simulink model "final_com_observer"  (R2017a)
settings: Solver=VariableStepAuto  StartTime=0.0  StopTime=15  RelTol=1e-3
values from neighbouring files (symbols this model uses):
  L = place (A',C',J_obs)    [principal.m]
undefined symbols (not defined in the file or in its folder): K_lqr
libraries: simulink x6
settings Model: Creator=dscat  LastModifiedBy=dscat

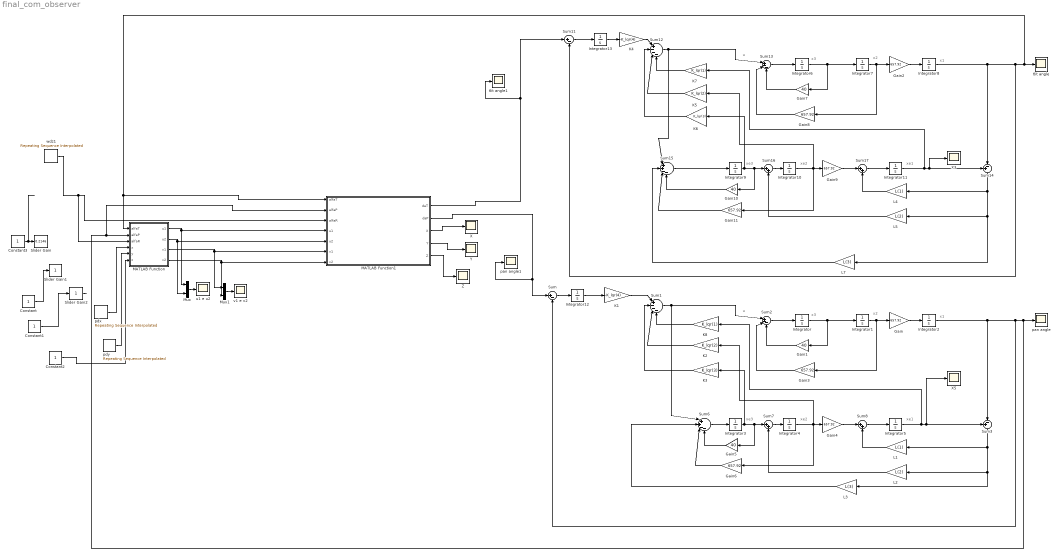
== system final_com_observer ==
  note: x2
  note: u
  note: xe1
  note: x1
  note: x3
  note: xe3
  note: xe2
  note: x2
  note: u
  note: xe1
  note: x1
  note: x3
  note: xe3
  note: xe2
  Constant{,1..3} (4 alike) : Constant
  Gain{,2..4,6,8..9,11} (8 alike) : Gain  Gain=657.92
  Gain{1,5,7,10} (4 alike) : Gain  Gain=40
  Integrator{,1..13} (14 alike) : Integrator
  K1 : Gain  Gain=-K_lqr(4)
  K2 : Gain  Gain=K_lqr(2)
  K3 : Gain  Gain=K_lqr(3)
  K4 : Gain  Gain=-K_lqr(4)
  K5 : Gain  Gain=K_lqr(2)
  K6 : Gain  Gain=K_lqr(3)
  K7 : Gain  Gain=K_lqr(1)
  K8 : Gain  Gain=K_lqr(1)
  L1 : Gain  Gain=L(1)
  L2 : Gain  Gain=L(2)
  L3 : Gain  Gain=L(3)
  L4 : Gain  Gain=L(1)
  L5 : Gain  Gain=L(2)
  L7 : Gain  Gain=L(3)
  MATLAB Function : MATLAB Function  TreatAsAtomicUnit=on
  MATLAB Function1 : MATLAB Function  TreatAsAtomicUnit=on
  Mux : Mux  Inputs=2
  Mux1 : Mux  Inputs=2
  Slider Gain : simulink/Math Operations/Slider Gain  gain=0.2146  low=-3.14  high=3.14
  Slider Gain1 : simulink/Math Operations/Slider Gain  gain=1  low=-5  high=5
  Slider Gain2 : simulink/Math Operations/Slider Gain  gain=1  low=-5  high=5
  Sum : Sum  Inputs=|+-
  Sum1 : Sum  Inputs=|+---
  Sum11 : Sum  Inputs=|+-
  Sum12 : Sum  Inputs=|+---
  Sum13 : Sum  Inputs=|+--
  Sum14 : Sum  Inputs=+-|
  Sum15 : Sum  Inputs=|++--
  Sum{7..8,16..17} (4 alike) : Sum  Inputs=|++
  Sum2 : Sum  Inputs=|+--
  Sum3 : Sum  Inputs=+-|
  Sum6 : Sum  Inputs=|++--
  X : Scope
  X3 : Scope
  X5 : Scope
  Y : Scope
  Z : Scope
  pan angle : Scope
  pan angle1 : Scope
  pdx : simulink/Sources/Repeating Sequence Interpolated  OutValues=pdx  TimeValues=t  LookUpMeth=Interpolation-Use End Values  tsamp=0.01  OutMin=[]  OutMax=[]  OutDataTypeStr=double  OutputDataTypeScalingMode=double  OutDataType=fixdt(0,8)  OutScaling=2^-10
  pdy : simulink/Sources/Repeating Sequence Interpolated  OutValues=pdy  TimeValues=t  LookUpMeth=Interpolation-Use End Values  tsamp=0.01  OutMin=[]  OutMax=[]  OutDataTypeStr=double  OutputDataTypeScalingMode=double  OutDataType=fixdt(0,8)  OutScaling=2^-10
  tlit angle : Scope
  tlit angle1 : Scope
  u1 e u2 : Scope
  v1 e v2 : Scope
  wdz1 : simulink/Sources/Repeating Sequence Interpolated  OutValues=wdz  TimeValues=t  LookUpMeth=Interpolation-Use End Values  tsamp=0.01  OutMin=[]  OutMax=[]  OutDataTypeStr=double  OutputDataTypeScalingMode=double  OutDataType=fixdt(0,8)  OutScaling=2^-10
  wires:
  MATLAB Function1/3(X) -> X/1
  MATLAB Function1/4(Y) -> Y/1
  MATLAB Function1/5(Z) -> Z/1
  Integrator8/1 -> Sum14/2, Sum11/2, tlit angle/1, MATLAB Function1/1(alfaT), MATLAB Function/1(alfaT)
  Integrator2/1 -> Sum3/2, Sum/2, pan angle/1, MATLAB Function1/2(alfaP), MATLAB Function/2(alfaP)
  Constant3/1 -> Slider Gain/1
  Constant1/1 -> Slider Gain2/1
  Mux1/1 -> v1 e v2/1
  Mux/1 -> u1 e u2/1
  Constant/1 -> Slider Gain1/1
  MATLAB Function/4(v2) -> MATLAB Function1/7(v2), Mux1/2
  MATLAB Function/1(u1) -> MATLAB Function1/4(u1), Mux/1
  MATLAB Function/3(v1) -> MATLAB Function1/6(v1), Mux1/1
  MATLAB Function/2(u2) -> MATLAB Function1/5(u2), Mux/2
  Gain5/1 -> Sum6/4
  Sum8/1 -> Integrator5/1
  Integrator4/1 -> K2/1, Gain6/1, Gain4/1
  L2/1 -> Sum7/2
  Sum7/1 -> Integrator4/1
  Gain4/1 -> Sum8/1
  Integrator3/1 -> Sum7/1, Gain5/1, K3/1
  K3/1 -> Sum1/2
  Sum/1 -> Integrator12/1
  L1/1 -> Sum8/2
  Gain6/1 -> Sum6/3
  Gain1/1 -> Sum2/3
  Integrator5/1 -> K8/1, X5/1, Sum3/1
  Gain3/1 -> Sum2/2
  L3/1 -> Sum6/2
  Sum3/1 -> L1/1, L2/1, L3/1
  MATLAB Function1/2(daP) -> pan angle1/1, Sum/1
  Integrator/1 -> Gain1/1, Integrator1/1
  Sum6/1 -> Integrator3/1
  Gain/1 -> Integrator2/1
  Integrator1/1 -> Gain3/1, Gain/1
  K2/1 -> Sum1/3
  Sum1/1 -> Sum2/1, Sum6/1
  Sum2/1 -> Integrator/1
  K1/1 -> Sum1/1
  Gain10/1 -> Sum15/4
  Sum17/1 -> Integrator11/1
  Integrator10/1 -> K5/1, Gain11/1, Gain9/1
  L5/1 -> Sum16/2
  Sum16/1 -> Integrator10/1
  Gain9/1 -> Sum17/1
  Integrator9/1 -> Sum16/1, Gain10/1, K6/1
  K6/1 -> Sum12/2
  Sum11/1 -> Integrator13/1
  L4/1 -> Sum17/2
  Gain11/1 -> Sum15/3
  Gain7/1 -> Sum13/3
  Integrator11/1 -> K7/1, X3/1, Sum14/1
  Gain8/1 -> Sum13/2
  Sum14/1 -> L4/1, L5/1, L7/1
  Integrator6/1 -> Gain7/1, Integrator7/1
  Gain2/1 -> Integrator8/1
  Integrator7/1 -> Gain8/1, Gain2/1
  K5/1 -> Sum12/3
  Sum12/1 -> Sum13/1, Sum15/1
  Sum13/1 -> Integrator6/1
  K4/1 -> Sum12/1
  Integrator13/1 -> K4/1
  K7/1 -> Sum12/4
  Sum15/1 -> Integrator9/1
  L7/1 -> Sum15/2
  K8/1 -> Sum1/4
  MATLAB Function1/1(daT) -> Sum11/1, tlit angle1/1
  Constant2/1 -> MATLAB Function/6(z)
  Integrator12/1 -> K1/1
  wdz1/1 -> MATLAB Function1/3(alfaR), MATLAB Function/3(alfaR)
  Slider Gain2/1 -> ?
  pdx/1 -> MATLAB Function/4(x)
  pdy/1 -> MATLAB Function/5(y)

== matlab function final_com_observer/MATLAB Function1 ==
  data: alfaT input; daT output; alfaP input; alfaR input; u1 input; u2 input; v1 input; v2 input; daP output; X output; Y output; Z output
function [daT, daP, X,Y,Z  ] = image2real( alfaT,alfaP,alfaR, u1,u2,v1,v2)
% daT -> Delta Alfa Tilt
% daP -> Delta Alfa Pan
% AlfaR -> Lido dos encoders


l = 0.15; %Tamanho do alvo (m) 
f = 664;

X = (l*(f*cos(alfaP-alfaR) - u2*sin(alfaP-alfaR))*(- cos(alfaP-alfaR)*sin(alfaP-alfaR)*f^2 + (u1 - cos(alfaP-alfaR)^2*(u1 + u2))*f + u1*u2*cos(alfaP-alfaR)*sin(alfaP-alfaR)))/(f*(u2*cos(alfaP-alfaR) + f*sin(alfaP-alfaR))*(u1 - u2));

%X = (l*(f*cos(alfaT) - v2*sin(alfaT))*(- cos(alfaT)*sin(alfaT)*f^2 + (v1 - cos(alfaT)^2*(v1 + v2))*f + v1*v2*cos(alfaT)*sin(alfaT)))/(f*(f*sin(alfaT) + v2*cos(alfaT))*(v1 - v2));

Y = -(l*(2*cos(alfaP-alfaR)*sin(alfaP-alfaR)*f^2 + (u1 + u2)*(2*cos(alfaP-alfaR)^2 - 1)*f - 2*u1*u2*cos(alfaP-alfaR)*sin(alfaP-alfaR)))/(2*f*(u1 - u2));

Z  = -(l*(2*cos(alfaT)*sin(alfaT)*f^2 + (v1 + v2)*(2*cos(alfaT)^2 - 1)*f - 2*v1*v2*cos(alfaT)*sin(alfaT)))/(2*f*(v1 - v2));
 
daP = double(atan(Y/X)+alfaR);
%daT = double(atan(Z/(sqrt((X)^2+(Y)^2))));
daT = double(atan(Z/X));

end

== matlab function final_com_observer/MATLAB Function ==
  data: alfaT input; u1 output; alfaP input; alfaR input; x input; y input; z input; u2 output; v1 output; v2 output
function [u1, u2, v1, v2] = real2image(alfaT,alfaP,alfaR,x,y,z)
L = 0.15;
f = 664;
u1 = f*(-sin(alfaP-alfaR)*(-x)+cos(alfaP-alfaR)*((L/2)-y))/((cos(alfaP-alfaR)*(-x)+sin(alfaP-alfaR)*((L/2)-y)));
u2 = f*(-sin(alfaP-alfaR)*(-x)+cos(alfaP-alfaR)*((-L/2)-y))/((cos(alfaP-alfaR)*(-x)+sin(alfaP-alfaR)*((-L/2)-y)));
v1 = f*(-sin(alfaT)*(-x)+cos(alfaT)*((L/2)-z))/((cos(alfaT)*(-x)+sin(alfaT)*((L/2)-z)));
v2 = f*(-sin(alfaT)*(-x)+cos(alfaT)*((-L/2)-z))/((cos(alfaT)*(-x)+sin(alfaT)*((-L/2)-z)));

end
